simulink model "model1"  (R2023b)
settings: Solver=ode4  StartTime=0.0  StopTime=5  FixedStep=Ts  RelTol=1e-3
values from neighbouring files (symbols this model uses):
  A_observer = A - L * C    [script_phase.m]
  B = [zeros(2,1) ... (first row only)    [script_phase.m]
  Kf = K    [script_phase.m]
  L = place(A', C', observer_poles)'    [script_phase.m]
  q10 = 0    [script_phase.m]
  q20 = pi    (= 3.14159265359)    [script_phase.m]
  X0 = [0; 0.95*pi; 0; 0]    [script_phase.m]
undefined symbols (not defined in the file or in its folder): Ph
settings Model: Creator=shahin  LastModifiedBy=bhatia32
settings DataIOCC: ReturnWorkspaceOutputs=off
settings OptimizationCC: ReuseModelBlockBuffer=off

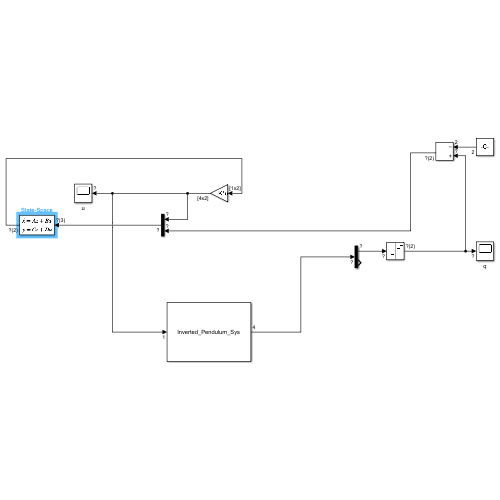
[thumbnail: Simulink's stored preview of the top-level diagram]
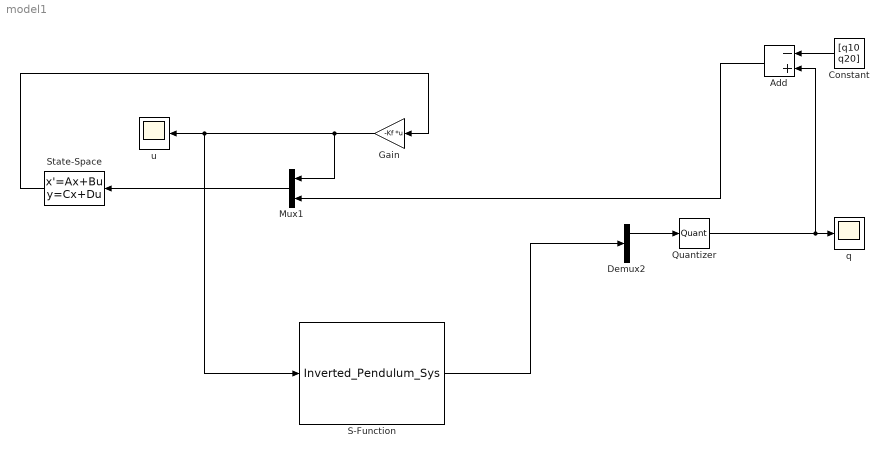
== system model1 ==
  Add : Sum  Inputs=-+
  Constant : Constant  Value="[q10  q20]"
  Demux2 : Demux  Outputs=2
  Gain : Gain  Gain=-Kf  Multiplication=Matrix(K*u)
  Mux1 : Mux  Inputs=2
  Quantizer : Quantizer  QuantizationInterval="[2*pi/2048  2*pi/2048]"
  S-Function : S-Function  FunctionName=Inverted_Pendulum_Sys  Parameters=X0,Ph  SFunctionDeploymentMode=off  EnableBusSupport=off
  State-Space : StateSpace  A=A_observer  B=[B L]  C=eye(4)  D=zeros(4,3)  InitialCondition=0
  q : Scope
  u : Scope
  wires:
  Demux2/1 -> Quantizer/1
  S-Function/1 -> Demux2/1
  Add/1 -> Mux1/2
  Quantizer/1 -> Add/2, q/1
  Constant/1 -> Add/1
  Gain/1 -> Mux1/1, S-Function/1, u/1
  Mux1/1 -> State-Space/1
  State-Space/1 -> Gain/1
